simulink model "prob_3"  (R2020b)
settings: Solver=VariableStepAuto  StartTime=0.0  StopTime=10.0  MaxStep=0.001  RelTol=1e-3
model workspace (MAT data in the model file):
  a0 = 1
  a1 = -0.1584
  b0 = 0.5792
  b1 = -0.5792
libraries: dspsrcs4 x1
settings Model: Creator=Lakshmi  LastModifiedBy=Lakshmi

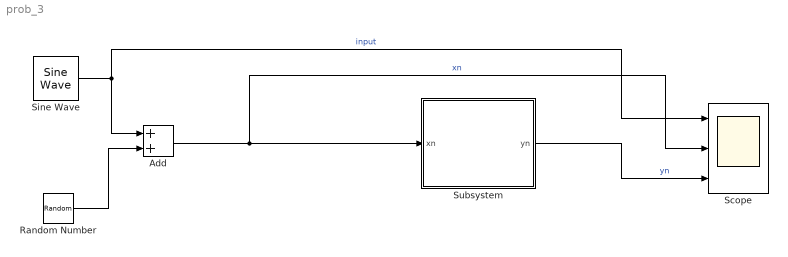
== system prob_3 ==
  Add : Sum
  Random Number : RandomNumber  SampleTime=0.1
  Scope : Scope  NumInputPorts=3
  Sine Wave : dspsrcs4/Sine Wave  Amplitude=2  Frequency=1000  Phase=0  SampleMode=Discrete  OutComplex=Real  CompMethod=Trigonometric fcn  TableSize=Speed  SampleTime=1/5000  SamplesPerFrame=1  ResetState=Restart at time zero  OutputFrames=off  dataType=double  wordLen=16  udDataType=sfix(16)  fracBitsMode=Best precision  numFracBits=15  OutDataTypeStr=double  LastOutDataTypeStr=double
  Subsystem : Subsystem
  wires:
  Add/1 -> Scope/2, Subsystem/1(xn)  "xn"
  Subsystem/1(yn) -> Scope/3  "yn"
  Random Number/1 -> Add/2
  Sine Wave/1 -> Add/1, Scope/1  "input"

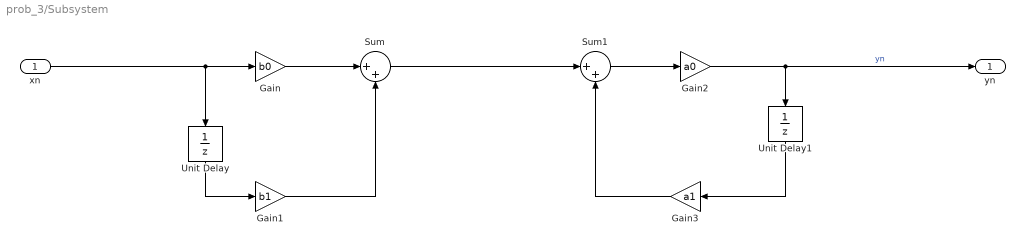
== system prob_3/Subsystem ==
  xn : Inport
  Gain : Gain  Gain=b0
  Gain1 : Gain  Gain=b1
  Gain2 : Gain  Gain=a0
  Gain3 : Gain  Gain=a1
  Sum : Sum  Inputs=|++
  Sum1 : Sum  Inputs=|++
  Unit Delay : UnitDelay  SampleTime=-1  HasFrameUpgradeWarning=on
  Unit Delay1 : UnitDelay  SampleTime=-1  HasFrameUpgradeWarning=on
  yn : Outport
  wires:
  Gain1/1 -> Sum/2
  Gain3/1 -> Sum1/2
  Unit Delay/1 -> Gain1/1
  Sum1/1 -> Gain2/1
  Unit Delay1/1 -> Gain3/1
  xn/1 -> Unit Delay/1, Gain/1
  Gain/1 -> Sum/1
  Sum/1 -> Sum1/1
  Gain2/1 -> yn/1, Unit Delay1/1  "yn"
